simulink model "ALU_tb"  (R2024b)
settings: Solver=VariableStepAuto  StartTime=0.0  StopTime=10.0  RelTol=1e-3
undefined symbols (not defined in the file): clockFrequency
settings Model: Creator=stefa  LastModifiedBy=stefano
settings RTWCC: GPUComputeCapability=3.5

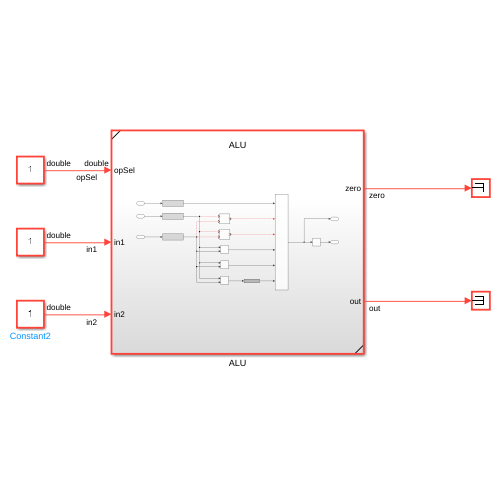
[thumbnail: Simulink's stored preview of the top-level diagram]
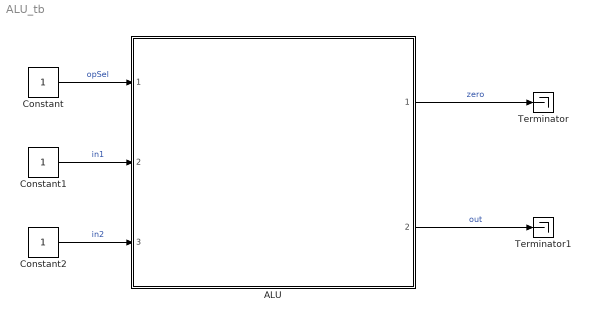
== system ALU_tb ==
  ALU : Subsystem  ReferencedSubsystem=ALU
  Constant : Constant  OutDataTypeStr=fixdt(0,4,0)  SampleTime=1/clockFrequency
  Constant1 : Constant  OutDataTypeStr=fixdt(0,32,0)  SampleTime=1/clockFrequency
  Constant2 : Constant  OutDataTypeStr=fixdt(0,32,0)  SampleTime=1/clockFrequency
  Terminator : Terminator
  Terminator1 : Terminator
  wires:
  ALU/1 -> Terminator/1  "zero"
  ALU/2 -> Terminator1/1  "out"
  Constant/1 -> ALU/1  "opSel"
  Constant1/1 -> ALU/2  "in1"
  Constant2/1 -> ALU/3  "in2"
